simulink model "P_2_1_b_Logisztikus_novekedes"  (R2021b)
settings: Solver=VariableStepAuto  StartTime=0.0  StopTime=75  RelTol=1e-3
settings Model: Creator=davidpaksi  LastModifiedBy=davidpaksi

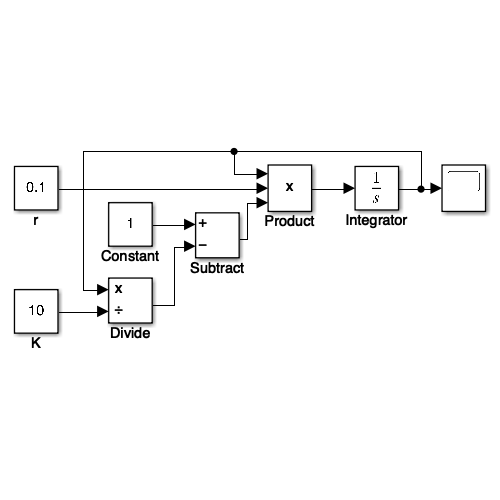
[thumbnail: Simulink's stored preview of the top-level diagram]
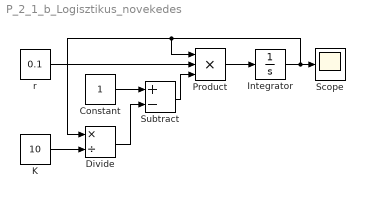
== system P_2_1_b_Logisztikus_novekedes ==
  "  Integrator  " : Integrator  InitialCondition=2
  " Constant " : Constant
  " Divide " : Product  Inputs=*/
  " Product " : Product  Inputs=3
  " Subtract " : Sum  Inputs=+-
  K : Constant  Value=10
  Scope : Scope
  r : Constant  Value=0.1
  wires:
  "  Integrator  "/1 -> Scope/1, " Divide "/1, " Product "/1
  " Product "/1 -> "  Integrator  "/1
  r/1 -> " Product "/2
  K/1 -> " Divide "/2
  " Constant "/1 -> " Subtract "/1
  " Divide "/1 -> " Subtract "/2
  " Subtract "/1 -> " Product "/3
